simulink model "untitled"  (Simulink 7.7)
settings: Solver=ode45  StartTime=0.0  StopTime=10.0  RelTol=1e-3
libraries: fuzblock x1
settings Model: Creator=ali  LastModifiedBy=ali

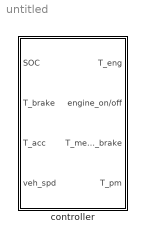
== system untitled ==
  controller : Subsystem

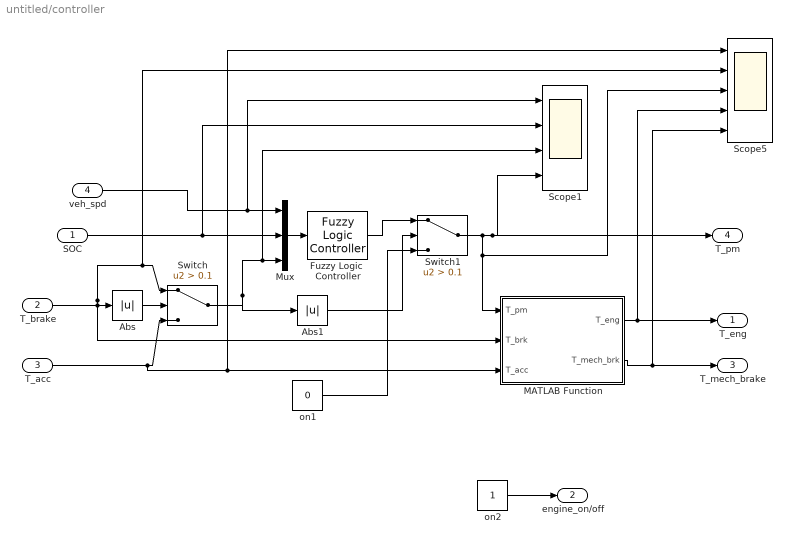
== system untitled/controller ==
  SOC : Inport
  T_brake : Inport  Port=2
  T_acc : Inport  Port=3
  veh_spd : Inport  Port=4
  Abs : Abs
  Abs1 : Abs
  Fuzzy Logic  Controller : fuzblock/Fuzzy Logic  Controller  SystemSampleTime=-1  fis=fuzy_controller1
  MATLAB Function : Stateflow chart  TreatAsAtomicUnit=on
  Mux : Mux  Inputs=3
  Scope1 : Scope  NumInputPorts=4
      settings: YMin=-2.5~41.5~-14000~0  YMax=17.5~45.5~1000~175  SaveName=ScopeData17  MaxDataPoints=500
  Scope5 : Scope  NumInputPorts=5
      settings: YMin=0~-350~-5~-5~-5  YMax=1000~500~5~5~5  SaveName=ScopeData21  MaxDataPoints=500
  Switch : Switch  Criteria=u2 > Threshold  Threshold=0.1
  Switch1 : Switch  Criteria=u2 > Threshold  Threshold=0.1
  on1 : Constant  Value=0
  on2 : Constant
  T_eng : Outport
  engine_on/off : Outport  Port=2
  T_mech_brake : Outport  Port=3
  T_pm : Outport  Port=4
  wires:
  on2/1 -> engine_on/off/1
  Mux/1 -> Fuzzy Logic  Controller/1
  veh_spd/1 -> Mux/1, Scope1/1
  SOC/1 -> Mux/2, Scope1/2
  Switch/1 -> Mux/3, Scope1/3, Abs1/1
  T_brake/1 -> Abs/1, MATLAB Function/2(T_brk), Switch/1, Scope5/2
  Abs/1 -> Switch/2
  T_acc/1 -> Switch/3, MATLAB Function/3(T_acc), Scope5/1
  MATLAB Function/1(T_eng) -> T_eng/1, Scope5/4
  MATLAB Function/2(T_mech_brk) -> T_mech_brake/1, Scope5/5
  Abs1/1 -> Switch1/2
  Fuzzy Logic  Controller/1 -> Switch1/1
  on1/1 -> Switch1/3
  Switch1/1 -> MATLAB Function/1(T_pm), Scope5/3, Scope1/4, T_pm/1

== matlab function controller/MATLAB Function ==
  data: T_pm input double; T_eng output double; T_brk input double; T_acc input double; T_mech_brk output double
function [T_eng,T_mech_brk] = fcn(T_pm,T_brk,T_acc)
if abs(T_brk)>0.1
    T_eng=0;
    T_mech_brk=min(0,T_brk-T_pm);
else
    T_mech_brk=0;
    T_eng=max(0,T_acc-T_pm);
end
end
